simulink model "pid_quadcopter"  (Simulink 7.9)
settings: Solver=ode4  StartTime=0.0  StopTime=t_end  FixedStep=.01  RelTol=1e-3
values from neighbouring files (symbols this model uses):
  C = [0 0 0]    [gen_smc_starter.m]    (also in pid_starter.m; sliding_starter.m)
  Cd = [0 0 0]    [gen_smc_starter.m]    (also in pid_starter.m; sliding_starter.m)
  g = 9.81    [gen_smc_starter.m]    (also in pid_starter.m; sliding_starter.m)
  I = [Ix Iy Iz]    [gen_smc_starter.m]    (also in pid_starter.m; sliding_starter.m)
  Kd = .95*[1 1]    [gen_smc_starter.m]    (also in pid_starter.m = [.01 .01 .6 .001 .001 0])
  Kf = 100    [gen_smc_starter.m]    (also in pid_starter.m; sliding_starter.m)
  Km = 1    [gen_smc_starter.m]    (also in pid_starter.m; sliding_starter.m)
  Kp = 1.0*[1 1]    [gen_smc_starter.m]    (also in pid_starter.m = [.01 .01 1 .035 .035 60])
  l = .25    (= 0.25)    [gen_smc_starter.m]    (also in pid_starter.m; sliding_starter.m)
  m = .5    (= 0.5)    [gen_smc_starter.m]    (also in pid_starter.m; sliding_starter.m)
  ref = [.1 0 .2 0 0 0]    [gen_smc_starter.m]    (also in pid_starter.m = [.1 -.1 .5 0 0 0]; sliding_starter.m = [0 2 1 0 0 0])
  step_time = [0 0 0]    [gen_smc_starter.m]    (also in pid_starter.m; sliding_starter.m)
  x0 = [0 0        0 0        .2 0        0 0        0 0        0 0        ]    [gen_smc_starter.m]    (also in pid_starter.m = [0 0        0 0        .1 0        0 0        0 0        0 0; sliding_starter.m = [0 0        0 0        .1 0        0 0        0 0        0 0)
settings Model: Creator=dwai  LastModifiedBy=dwai
settings DataIOCC: LimitDataPoints=off

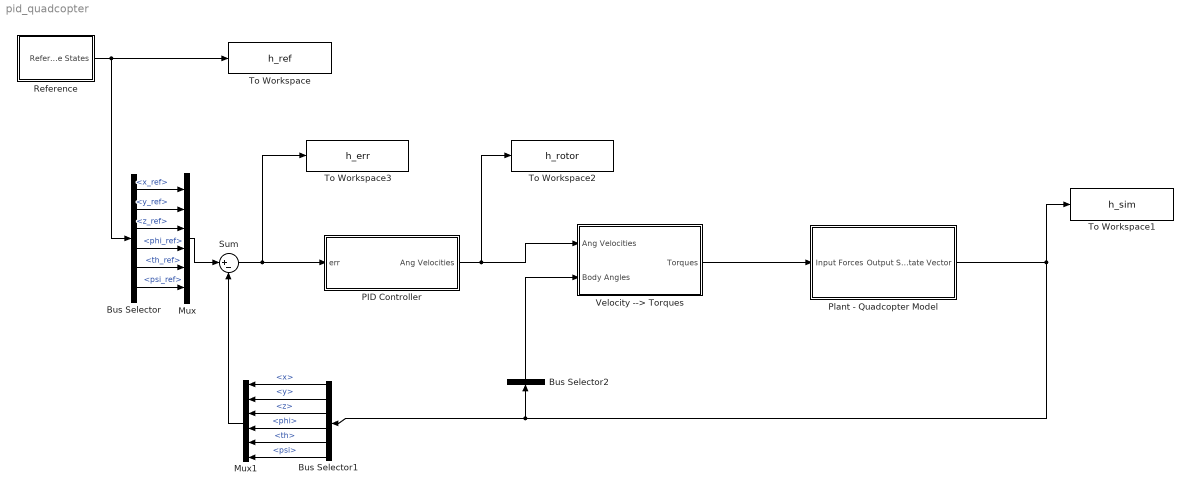
== system pid_quadcopter ==
  Bus Selector : BusSelector  OutputSignals=x_ref,y_ref,z_ref,phi_ref,th_ref,psi_ref
  Bus Selector1 : BusSelector  OutputSignals=x,y,z,phi,th,psi
  Bus Selector2 : BusSelector  OutputSignals=phi,th,psi  OutputAsBus=on
  Mux : Mux  Inputs=6
  Mux1 : Mux  Inputs=6
  PID Controller : Subsystem
  Plant - Quadcopter Model : Subsystem
  Reference : Subsystem
  Sum : Sum  Inputs=|+-
  To Workspace : ToWorkspace  VariableName=h_ref  SampleTime=-1  SaveFormat=Timeseries
  To Workspace1 : ToWorkspace  VariableName=h_sim  SampleTime=-1  SaveFormat=Timeseries
  To Workspace2 : ToWorkspace  VariableName=h_rotor  SampleTime=-1  SaveFormat=Timeseries
  To Workspace3 : ToWorkspace  VariableName=h_err  SampleTime=-1  SaveFormat=Timeseries
  Velocity --> Torques : Subsystem
  wires:
  Velocity --> Torques/1(Torques) -> Plant - Quadcopter Model/1(Input Forces)
  Plant - Quadcopter Model/1(Output State Vector) -> To Workspace1/1, Bus Selector1/1, Bus Selector2/1
  Reference/1(Reference States) -> Bus Selector/1, To Workspace/1
  Bus Selector/1 -> Mux/1  "<x_ref>"
  Bus Selector/2 -> Mux/2  "<y_ref>"
  Bus Selector/3 -> Mux/3  "<z_ref>"
  Bus Selector1/1 -> Mux1/1  "<x>"
  Bus Selector1/2 -> Mux1/2  "<y>"
  Bus Selector1/3 -> Mux1/3  "<z>"
  Mux/1 -> Sum/1
  Mux1/1 -> Sum/2
  Sum/1 -> PID Controller/1(err), To Workspace3/1
  PID Controller/1(Ang Velocities) -> Velocity --> Torques/1(Ang Velocities), To Workspace2/1
  Bus Selector2/1 -> Velocity --> Torques/2(Body Angles)
  Bus Selector/4 -> Mux/4  "<phi_ref>"
  Bus Selector/5 -> Mux/5  "<th_ref>"
  Bus Selector/6 -> Mux/6  "<psi_ref>"
  Bus Selector1/4 -> Mux1/4  "<phi>"
  Bus Selector1/5 -> Mux1/5  "<th>"
  Bus Selector1/6 -> Mux1/6  "<psi>"

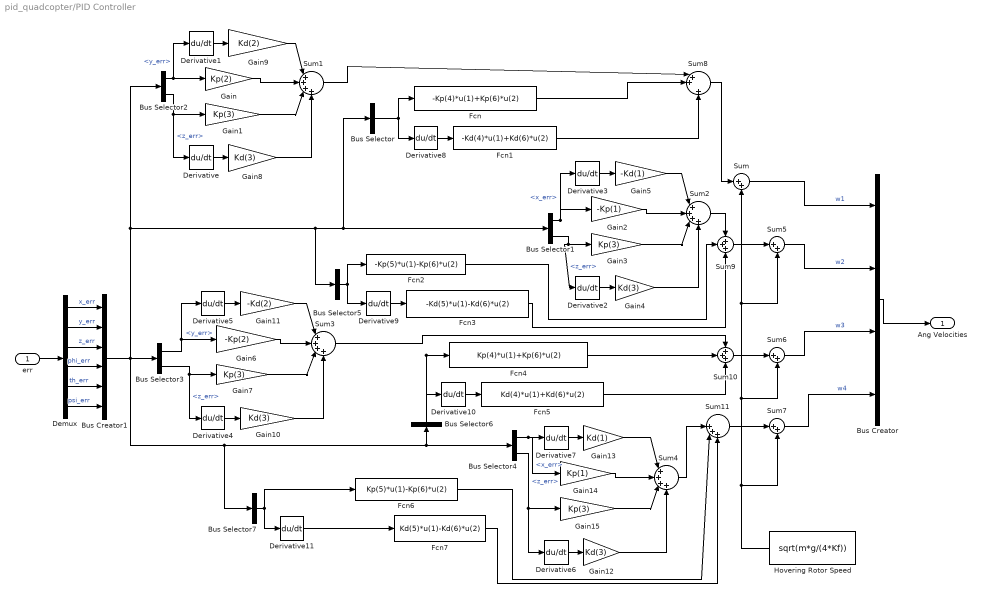
== system pid_quadcopter/PID Controller ==
  err : Inport
  Bus Creator : BusCreator
  Bus Creator1 : BusCreator  Inputs=6
  Bus Selector : BusSelector  OutputSignals=phi_err,psi_err  OutputAsBus=on
  Bus Selector1 : BusSelector  OutputSignals=x_err,z_err
  Bus Selector2 : BusSelector  OutputSignals=y_err,z_err
  Bus Selector3 : BusSelector  OutputSignals=y_err,z_err
  Bus Selector4 : BusSelector  OutputSignals=x_err,z_err
  Bus Selector5 : BusSelector  OutputSignals=th_err,psi_err  OutputAsBus=on
  Bus Selector6 : BusSelector  OutputSignals=phi_err,psi_err  OutputAsBus=on
  Bus Selector7 : BusSelector  OutputSignals=th_err,psi_err  OutputAsBus=on
  Demux : Demux  Outputs=6
  Derivative{,1..11} (12 alike) : Derivative
  Fcn : Fcn  Expr=-Kp(4)*u(1)+Kp(6)*u(2)
  Fcn1 : Fcn  Expr=-Kd(4)*u(1)+Kd(6)*u(2)
  Fcn2 : Fcn  Expr=-Kp(5)*u(1)-Kp(6)*u(2)
  Fcn3 : Fcn  Expr=-Kd(5)*u(1)-Kd(6)*u(2)
  Fcn4 : Fcn  Expr=Kp(4)*u(1)+Kp(6)*u(2)
  Fcn5 : Fcn  Expr=Kd(4)*u(1)+Kd(6)*u(2)
  Fcn6 : Fcn  Expr=Kp(5)*u(1)-Kp(6)*u(2)
  Fcn7 : Fcn  Expr=Kd(5)*u(1)-Kd(6)*u(2)
  Gain : Gain  Gain=Kp(2)
  Gain{1,3,7,15} (4 alike) : Gain  Gain=Kp(3)
  Gain{4,8,10,12} (4 alike) : Gain  Gain=Kd(3)
  Gain11 : Gain  Gain=-Kd(2)
  Gain13 : Gain  Gain=Kd(1)
  Gain14 : Gain  Gain=Kp(1)
  Gain2 : Gain  Gain=-Kp(1)
  Gain5 : Gain  Gain=-Kd(1)
  Gain6 : Gain  Gain=-Kp(2)
  Gain9 : Gain  Gain=Kd(2)
  Hovering Rotor Speed : Constant  Value=sqrt(m*g/(4*Kf))
  Sum{,5..7} (4 alike) : Sum  Inputs=|++
  Sum{1..4} (4 alike) : Sum  Inputs=|++++
  Sum10 : Sum  Inputs=+++
  Sum11 : Sum  Inputs=||+++
  Sum8 : Sum  Inputs=|++|+
  Sum9 : Sum  Inputs=+++
  Ang Velocities : Outport
  wires:
  Bus Creator/1 -> Ang Velocities/1
  Bus Creator1/1 -> Bus Selector2/1, Bus Selector1/1, Bus Selector/1, Bus Selector5/1, Bus Selector3/1, Bus Selector4/1, Bus Selector6/1, Bus Selector7/1
  Gain1/1 -> Sum1/3
  Bus Selector2/2 -> Gain1/1, Derivative/1  "<z_err>"
  Bus Selector2/1 -> Gain/1, Derivative1/1  "<y_err>"
  Demux/3 -> Bus Creator1/3  "z_err"
  Demux/1 -> Bus Creator1/1  "x_err"
  Demux/2 -> Bus Creator1/2  "y_err"
  err/1 -> Demux/1
  Sum7/1 -> Bus Creator/4  "w4"
  Sum6/1 -> Bus Creator/3  "w3"
  Sum5/1 -> Bus Creator/2  "w2"
  Sum/1 -> Bus Creator/1  "w1"
  Derivative/1 -> Gain8/1
  Gain/1 -> Sum1/2
  Derivative1/1 -> Gain9/1
  Gain9/1 -> Sum1/1
  Gain8/1 -> Sum1/4
  Gain3/1 -> Sum2/3
  Derivative2/1 -> Gain4/1
  Gain2/1 -> Sum2/2
  Derivative3/1 -> Gain5/1
  Gain5/1 -> Sum2/1
  Gain4/1 -> Sum2/4
  Bus Selector1/1 -> Gain2/1, Derivative3/1  "<x_err>"
  Bus Selector1/2 -> Gain3/1, Derivative2/1  "<z_err>"
  Gain7/1 -> Sum3/3
  Derivative4/1 -> Gain10/1
  Gain6/1 -> Sum3/2
  Derivative5/1 -> Gain11/1
  Gain11/1 -> Sum3/1
  Gain10/1 -> Sum3/4
  Bus Selector3/1 -> Derivative5/1, Gain6/1  "<y_err>"
  Bus Selector3/2 -> Gain7/1, Derivative4/1  "<z_err>"
  Gain15/1 -> Sum4/3
  Derivative6/1 -> Gain12/1
  Gain14/1 -> Sum4/2
  Derivative7/1 -> Gain13/1
  Gain13/1 -> Sum4/1
  Gain12/1 -> Sum4/4
  Bus Selector4/2 -> Derivative6/1, Gain15/1  "<z_err>"
  Hovering Rotor Speed/1 -> Sum/2, Sum5/2, Sum6/2, Sum7/2
  Demux/4 -> Bus Creator1/4  "phi_err"
  Demux/5 -> Bus Creator1/5  "th_err"
  Demux/6 -> Bus Creator1/6  "psi_err"
  Bus Selector/1 -> Fcn/1, Derivative8/1
  Derivative8/1 -> Fcn1/1
  Fcn1/1 -> Sum8/3
  Sum8/1 -> Sum/1
  Bus Selector5/1 -> Fcn2/1, Derivative9/1
  Derivative9/1 -> Fcn3/1
  Sum9/1 -> Sum5/1
  Sum2/1 -> Sum9/1
  Fcn3/1 -> Sum9/3
  Fcn2/1 -> Sum9/2
  Bus Selector6/1 -> Fcn4/1, Derivative10/1
  Derivative10/1 -> Fcn5/1
  Sum3/1 -> Sum10/1
  Fcn4/1 -> Sum10/2
  Fcn5/1 -> Sum10/3
  Sum10/1 -> Sum6/1
  Bus Selector4/1 -> Gain14/1, Derivative7/1  "<x_err>"
  Bus Selector7/1 -> Fcn6/1, Derivative11/1
  Derivative11/1 -> Fcn7/1
  Sum4/1 -> Sum11/1
  Fcn7/1 -> Sum11/3
  Fcn6/1 -> Sum11/2
  Sum11/1 -> Sum7/1
  Fcn/1 -> Sum8/2
  Sum1/1 -> Sum8/1

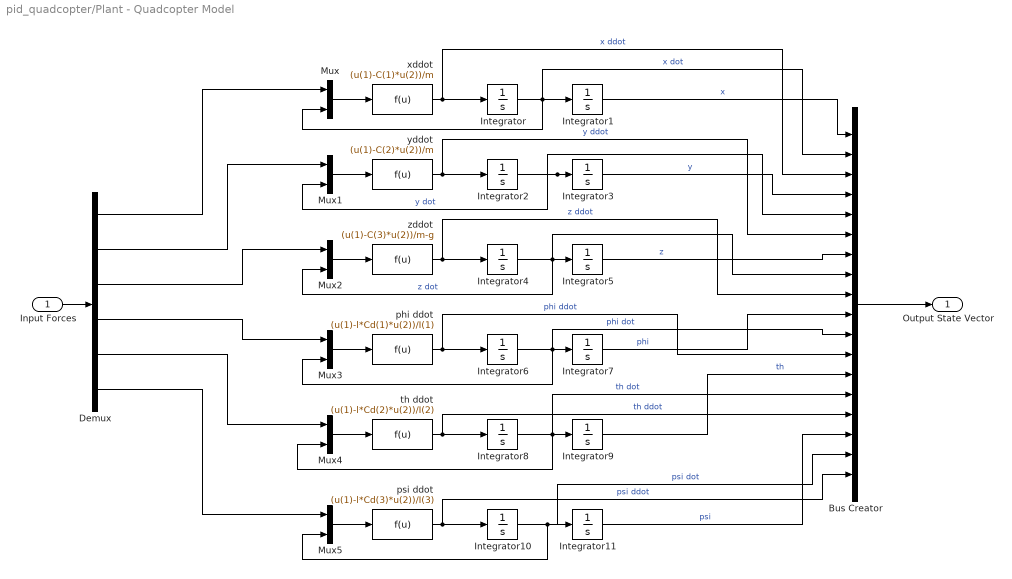
== system pid_quadcopter/Plant - Quadcopter Model ==
  Input Forces : Inport
  Bus Creator : BusCreator  Inputs=18
  Demux : Demux  Outputs=6
  Integrator : Integrator  InitialCondition=x0(2)
  Integrator1 : Integrator  InitialCondition=x0(1)
  Integrator10 : Integrator  InitialCondition=x0(12)
  Integrator11 : Integrator  InitialCondition=x0(11)
  Integrator2 : Integrator  InitialCondition=x0(4)
  Integrator3 : Integrator  InitialCondition=x0(3)
  Integrator4 : Integrator  InitialCondition=x0(6)
  Integrator5 : Integrator  InitialCondition=x0(5)
  Integrator6 : Integrator  InitialCondition=x0(8)
  Integrator7 : Integrator  InitialCondition=x0(7)
  Integrator8 : Integrator  InitialCondition=x0(10)
  Integrator9 : Integrator  InitialCondition=x0(9)
  Mux{,1..5} (6 alike) : Mux  Inputs=2
  phi ddot : Fcn  Expr=(u(1)-l*Cd(1)*u(2))/I(1)
  psi ddot : Fcn  Expr=(u(1)-l*Cd(3)*u(2))/I(3)
  th ddot : Fcn  Expr=(u(1)-l*Cd(2)*u(2))/I(2)
  xddot : Fcn  Expr=(u(1)-C(1)*u(2))/m
  yddot : Fcn  Expr=(u(1)-C(2)*u(2))/m
  zddot : Fcn  Expr=(u(1)-C(3)*u(2))/m-g
  Output State Vector : Outport
  wires:
  Demux/6 -> Mux5/1
  Demux/5 -> Mux4/1
  Demux/4 -> Mux3/1
  Demux/3 -> Mux2/1
  Demux/2 -> Mux1/1
  Demux/1 -> Mux/1
  Input Forces/1 -> Demux/1
  Integrator11/1 -> Bus Creator/16  "psi"
  Integrator9/1 -> Bus Creator/13  "th"
  Integrator7/1 -> Bus Creator/10  "phi"
  Integrator5/1 -> Bus Creator/7  "z"
  Integrator3/1 -> Bus Creator/4  "y"
  Integrator1/1 -> Bus Creator/1  "x"
  Integrator10/1 -> Integrator11/1, Mux5/2, Bus Creator/17  "psi dot"
  psi ddot/1 -> Integrator10/1, Bus Creator/18  "psi ddot"
  Mux5/1 -> psi ddot/1
  Integrator8/1 -> Integrator9/1, Mux4/2, Bus Creator/14  "th dot"
  th ddot/1 -> Integrator8/1, Bus Creator/15  "th ddot"
  Mux4/1 -> th ddot/1
  Integrator6/1 -> Integrator7/1, Mux3/2, Bus Creator/11  "phi dot"
  phi ddot/1 -> Integrator6/1, Bus Creator/12  "phi ddot"
  Mux3/1 -> phi ddot/1
  Integrator4/1 -> Integrator5/1, Mux2/2, Bus Creator/8  "z dot"
  zddot/1 -> Integrator4/1, Bus Creator/9  "z ddot"
  Mux2/1 -> zddot/1
  Integrator2/1 -> Integrator3/1, Mux1/2, Bus Creator/5  "y dot"
  yddot/1 -> Integrator2/1, Bus Creator/6  "y ddot"
  Mux1/1 -> yddot/1
  Integrator/1 -> Integrator1/1, Mux/2, Bus Creator/2  "x dot"
  xddot/1 -> Integrator/1, Bus Creator/3  "x ddot"
  Mux/1 -> xddot/1
  Bus Creator/1 -> Output State Vector/1

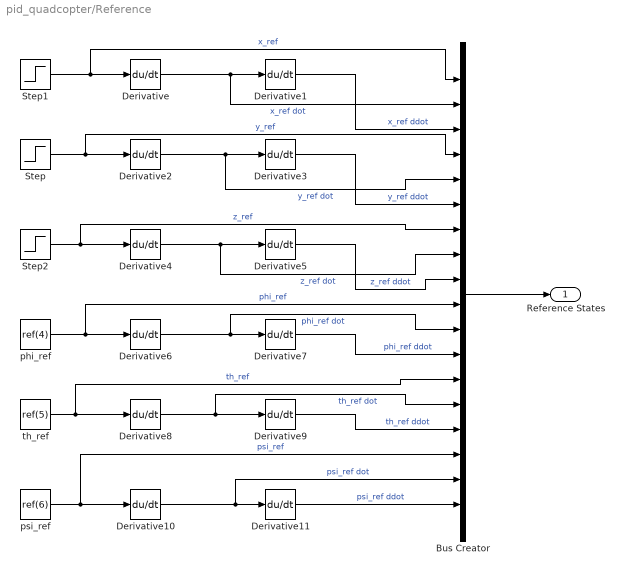
== system pid_quadcopter/Reference ==
  Bus Creator : BusCreator  Inputs=18
  Derivative{,1..11} (12 alike) : Derivative
  Step : Step  Time=step_time(2)  After=ref(2)  SampleTime=0
  Step1 : Step  Time=step_time(1)  After=ref(1)  SampleTime=0
  Step2 : Step  Time=step_time(3)  After=ref(3)  SampleTime=0
  phi_ref : Constant  Value=ref(4)
  psi_ref : Constant  Value=ref(6)
  th_ref : Constant  Value=ref(5)
  Reference States : Outport
  wires:
  Derivative/1 -> Derivative1/1, Bus Creator/2  "x_ref dot"
  Derivative2/1 -> Derivative3/1, Bus Creator/5  "y_ref dot"
  Step2/1 -> Derivative4/1, Bus Creator/7  "z_ref"
  Derivative4/1 -> Derivative5/1, Bus Creator/8  "z_ref dot"
  phi_ref/1 -> Derivative6/1, Bus Creator/10  "phi_ref"
  Derivative6/1 -> Derivative7/1, Bus Creator/11  "phi_ref dot"
  th_ref/1 -> Derivative8/1, Bus Creator/13  "th_ref"
  Derivative8/1 -> Derivative9/1, Bus Creator/14  "th_ref dot"
  psi_ref/1 -> Derivative10/1, Bus Creator/16  "psi_ref"
  Derivative10/1 -> Derivative11/1, Bus Creator/17  "psi_ref dot"
  Derivative1/1 -> Bus Creator/3  "x_ref ddot"
  Derivative3/1 -> Bus Creator/6  "y_ref ddot"
  Derivative5/1 -> Bus Creator/9  "z_ref ddot"
  Derivative7/1 -> Bus Creator/12  "phi_ref ddot"
  Derivative9/1 -> Bus Creator/15  "th_ref ddot"
  Derivative11/1 -> Bus Creator/18  "psi_ref ddot"
  Bus Creator/1 -> Reference States/1
  Step/1 -> Derivative2/1, Bus Creator/4  "y_ref"
  Step1/1 -> Derivative/1, Bus Creator/1  "x_ref"

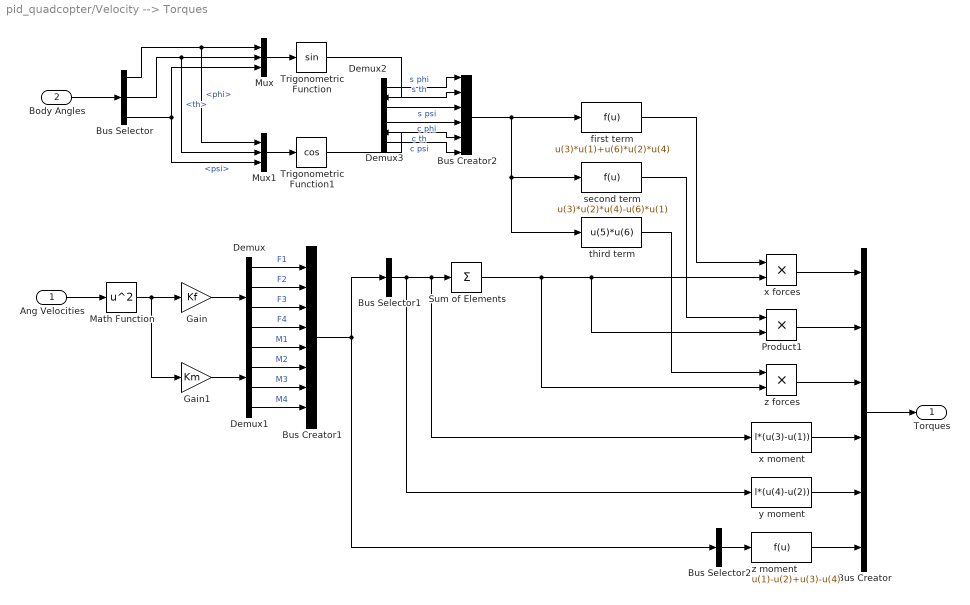
== system pid_quadcopter/Velocity --> Torques ==
  Ang Velocities : Inport
  Body Angles : Inport  Port=2
  Bus Creator : BusCreator  Inputs=6
  Bus Creator1 : BusCreator  Inputs=8
  Bus Creator2 : BusCreator  Inputs=6
  Bus Selector : BusSelector  OutputSignals=phi,th,psi
  Bus Selector1 : BusSelector  OutputSignals=F1,F2,F3,F4  OutputAsBus=on
  Bus Selector2 : BusSelector  OutputSignals=M1,M2,M3,M4  OutputAsBus=on
  Demux : Demux
  Demux1 : Demux
  Demux2 : Demux  Outputs=3
  Demux3 : Demux  Outputs=3
  Gain : Gain  Gain=Kf
  Gain1 : Gain  Gain=Km
  Math Function : Math  Operator=square  SaturateOnIntegerOverflow=on
  Mux : Mux  Inputs=3
  Mux1 : Mux  Inputs=3
  Product1 : Product  RndMeth=Zero
  Sum of Elements : Sum  Inputs=+
  Trigonometric Function : Trigonometry
  Trigonometric Function1 : Trigonometry  Operator=cos
  first term : Fcn  Expr=u(3)*u(1)+u(6)*u(2)*u(4)
  second term : Fcn  Expr=u(3)*u(2)*u(4)-u(6)*u(1)
  third term : Fcn  Expr=u(5)*u(6)
  x forces : Product  RndMeth=Zero
  x moment : Fcn  Expr=l*(u(3)-u(1))
  y moment : Fcn  Expr=l*(u(4)-u(2))
  z forces : Product  RndMeth=Zero
  z moment : Fcn  Expr=u(1)-u(2)+u(3)-u(4)
  Torques : Outport
  wires:
  Bus Creator/1 -> Torques/1
  Ang Velocities/1 -> Math Function/1
  Math Function/1 -> Gain/1, Gain1/1
  Gain/1 -> Demux/1
  Gain1/1 -> Demux1/1
  Demux1/4 -> Bus Creator1/8  "M4"
  Demux1/3 -> Bus Creator1/7  "M3"
  Demux1/2 -> Bus Creator1/6  "M2"
  Demux1/1 -> Bus Creator1/5  "M1"
  Demux/4 -> Bus Creator1/4  "F4"
  Demux/3 -> Bus Creator1/3  "F3"
  Demux/2 -> Bus Creator1/2  "F2"
  Demux/1 -> Bus Creator1/1  "F1"
  Body Angles/1 -> Bus Selector/1
  Bus Selector/3 -> Mux/3, Mux1/3  "<psi>"
  Bus Selector/2 -> Mux/2, Mux1/2  "<th>"
  Bus Selector/1 -> Mux/1, Mux1/1  "<phi>"
  Mux/1 -> Trigonometric Function/1
  Mux1/1 -> Trigonometric Function1/1
  Trigonometric Function/1 -> Demux2/1
  Trigonometric Function1/1 -> Demux3/1
  Demux2/1 -> Bus Creator2/1  "s phi"
  Demux2/2 -> Bus Creator2/2  "s th"
  Demux2/3 -> Bus Creator2/3  "s psi"
  Demux3/1 -> Bus Creator2/4  "c phi"
  Demux3/2 -> Bus Creator2/5  "c th"
  Demux3/3 -> Bus Creator2/6  "c psi"
  Bus Creator2/1 -> first term/1, second term/1, third term/1
  Bus Creator1/1 -> Bus Selector1/1, Bus Selector2/1
  Bus Selector1/1 -> Sum of Elements/1, x moment/1, y moment/1
  x forces/1 -> Bus Creator/1
  first term/1 -> x forces/1
  Sum of Elements/1 -> z forces/2, x forces/2, Product1/2
  second term/1 -> Product1/1
  third term/1 -> z forces/1
  Product1/1 -> Bus Creator/2
  z forces/1 -> Bus Creator/3
  z moment/1 -> Bus Creator/6
  Bus Selector2/1 -> z moment/1
  x moment/1 -> Bus Creator/4
  y moment/1 -> Bus Creator/5
